simulink model "motor_ac"  (R2022b)
settings: Solver=VariableStepAuto  StartTime=0.0  StopTime=0.05  RelTol=1e-9  AbsTol=1e-9
values from neighbouring files (symbols this model uses):
  a1 = 1    [loop_sim.m]    (also in var_motor.m)
  a2 = 0.05    [loop_sim.m]    (also in sim_motor.m = a2s(i); var_motor.m)
  a3 = 0.02    [loop_sim.m]    (also in sim_motor.m = a3s(i); var_motor.m)
  Bm = 80e-6    (= 8e-05)    [loop_sim.m]    (also in var_motor.m)
  Jm = 40e-6    (= 4e-05)    [loop_sim.m]    (also in var_motor.m)
  Lls = 0.2e-3    (= 0.0002)    [loop_sim.m]    (also in var_motor.m)
  Lmb = 1.8e-3    (= 0.0018)    [loop_sim.m]    (also in var_motor.m)
  P = 4    [loop_sim.m]    (also in var_motor.m)
  psim = 0.1    [loop_sim.m]    (also in sim_motor.m = PSIs(i); var_motor.m)
  rs = 1    [loop_sim.m]    (also in sim_motor.m = RSs(i); var_motor.m)
  TL = 0.5    [loop_sim.m]    (also in var_motor.m = 0.1)
  TL0 = 0.5    [loop_sim.m]    (also in var_motor.m = 0.1)
  uM = 50    [loop_sim.m]    (also in var_motor.m)
settings Model: Creator=yodap  LastModifiedBy=andre
settings OptimizationCC: ReuseModelBlockBuffer=on

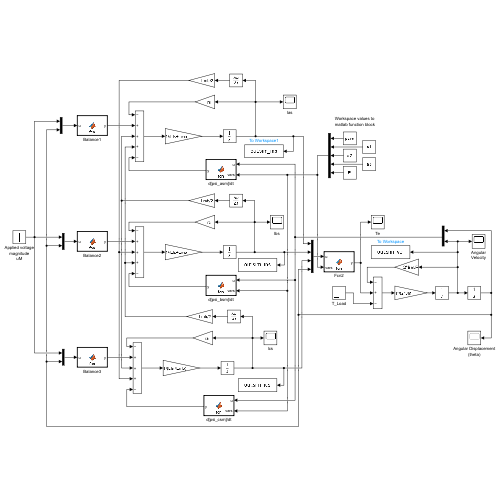
[thumbnail: Simulink's stored preview of the top-level diagram]
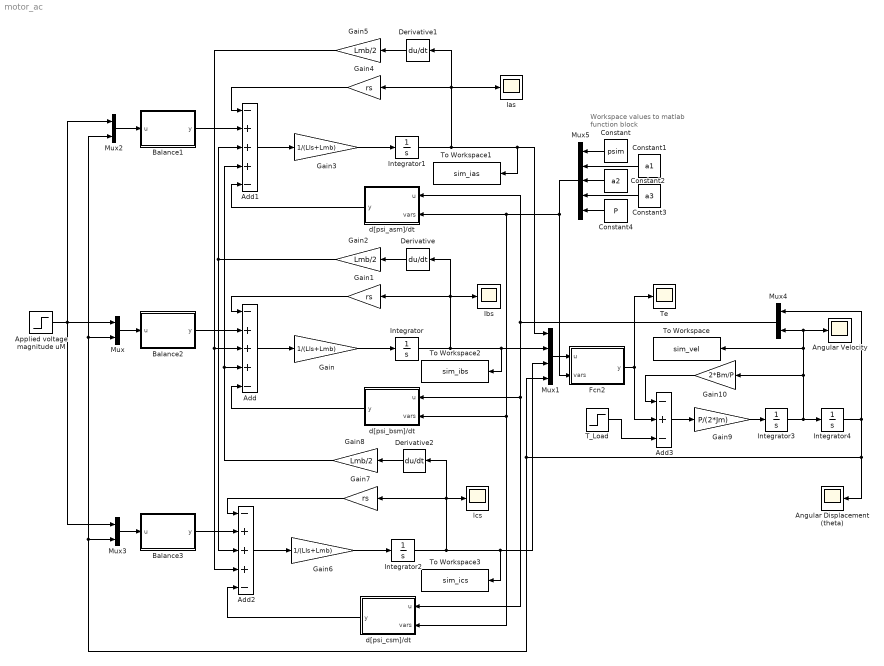
== system motor_ac ==
  note: Workspace values to
      | matlab function block
  Add : Sum  Inputs=-+++-
  Add1 : Sum  Inputs=-+++-
  Add2 : Sum  Inputs=-+++-
  Add3 : Sum  Inputs=-+-
  Angular Velocity : Scope
  Angular Displacement (theta) : Scope
  Applied voltage magnitude uM : Step  Time=0  After=uM  SampleTime=0
  Balance1 : MATLAB Function  TreatAsAtomicUnit=on
  Balance2 : MATLAB Function  TreatAsAtomicUnit=on
  Balance3 : MATLAB Function  TreatAsAtomicUnit=on
  Constant : Constant  Value=psim
  Constant1 : Constant  Value=a1
  Constant2 : Constant  Value=a2
  Constant3 : Constant  Value=a3
  Constant4 : Constant  Value=P
  Derivative : Derivative
  Derivative1 : Derivative
  Derivative2 : Derivative
  Fcn2 : MATLAB Function  TreatAsAtomicUnit=on
  Gain : Gain  Gain=1/(Lls+Lmb)
  Gain1 : Gain  Gain=rs
  Gain10 : Gain  Gain=2*Bm/P
  Gain2 : Gain  Gain=Lmb/2
  Gain3 : Gain  Gain=1/(Lls+Lmb)
  Gain4 : Gain  Gain=rs
  Gain5 : Gain  Gain=Lmb/2
  Gain6 : Gain  Gain=1/(Lls+Lmb)
  Gain7 : Gain  Gain=rs
  Gain8 : Gain  Gain=Lmb/2
  Gain9 : Gain  Gain=P/(2*Jm)
  Ias : Scope
  Ibs : Scope
  Integrator{,1..4} (5 alike) : Integrator
  Mux{,2..4} (4 alike) : Mux  Inputs=2
  Mux1 : Mux
  Mux5 : Mux  Inputs=5
  T_Load : Step  Time=0.025  Before=TL0  After=TL  SampleTime=0
  Te : Scope
  To Workspace : ToWorkspace  VariableName=sim_vel  SaveFormat=Timeseries  SampleTime=-1
  To Workspace1 : ToWorkspace  VariableName=sim_ias  SaveFormat=Timeseries  SampleTime=-1
  To Workspace2 : ToWorkspace  VariableName=sim_ibs  SaveFormat=Timeseries  SampleTime=-1
  To Workspace3 : ToWorkspace  VariableName=sim_ics  SaveFormat=Timeseries  SampleTime=-1
  d[psi_asm]/dt : MATLAB Function  TreatAsAtomicUnit=on
  d[psi_bsm]/dt : MATLAB Function  TreatAsAtomicUnit=on
  d[psi_csm]/dt : MATLAB Function  TreatAsAtomicUnit=on
  lcs : Scope
  wires:
  Mux/1 -> Balance2/1(u)
  Applied voltage magnitude uM/1 -> Mux3/1, Mux2/1, Mux/1
  Add/1 -> Gain/1
  Gain/1 -> Integrator/1
  Gain1/1 -> Add/1
  Integrator/1 -> To Workspace2/1, Mux1/2, Ibs/1, Gain1/1, Derivative/1
  Derivative/1 -> Gain2/1
  Gain3/1 -> Integrator1/1
  Add1/1 -> Gain3/1
  Gain4/1 -> Add1/1
  Derivative1/1 -> Gain5/1
  Integrator1/1 -> Gain4/1, Ias/1, Derivative1/1, To Workspace1/1, Mux1/1
  Gain2/1 -> Add2/3, Add1/3
  Balance1/1(y) -> Add1/2
  Mux2/1 -> Balance1/1(u)
  Derivative2/1 -> Gain8/1
  Integrator2/1 -> Derivative2/1, Gain7/1, lcs/1, To Workspace3/1, Mux1/3
  d[psi_csm]/dt/1(y) -> Add2/5
  Gain7/1 -> Add2/1
  Gain6/1 -> Integrator2/1
  Add2/1 -> Gain6/1
  Gain8/1 -> Add1/4, Add/4
  Gain5/1 -> Add2/4, Add/3
  T_Load/1 -> Add3/3
  Add3/1 -> Gain9/1
  Gain9/1 -> Integrator3/1
  Gain10/1 -> Add3/1
  Integrator3/1 -> Mux4/2, Angular Velocity/1, To Workspace/1, Gain10/1, Integrator4/1
  Mux4/1 -> d[psi_csm]/dt/1(u), d[psi_bsm]/dt/1(u), d[psi_asm]/dt/1(u)
  Integrator4/1 -> Mux2/2, Mux/2, Mux3/2, Mux1/4, Angular Displacement (theta)/1, Mux4/1
  Mux1/1 -> Fcn2/1(u)
  Fcn2/1(y) -> Te/1, Add3/2
  Balance2/1(y) -> Add/2
  Mux3/1 -> Balance3/1(u)
  Balance3/1(y) -> Add2/2
  d[psi_bsm]/dt/1(y) -> Add/5
  d[psi_asm]/dt/1(y) -> Add1/5
  Constant1/1 -> Mux5/2
  Constant2/1 -> Mux5/3
  Constant3/1 -> Mux5/4
  Constant/1 -> Mux5/1
  Mux5/1 -> Fcn2/2(vars), d[psi_csm]/dt/2(vars), d[psi_bsm]/dt/2(vars), d[psi_asm]/dt/2(vars)
  Constant4/1 -> Mux5/5

== matlab function motor_ac/Fcn2 ==
  data: u input; y output; vars input
function y = fcn(u,vars)

psim = vars(1);
a1 = vars(2);
a2 = vars(3);
a3 = vars(4);
P = vars(5);

y = P*psim*(u(1)*cos(u(4))*(a1+3*a2*(sin(u(4)))^2+5*a3*(sin(u(4)))^4)+u(2)*cos(u(4)+2*pi/3)*(a1+3*a2*(sin(u(4)+2*pi/3))^2+5*a3*(sin(u(4)+2*pi/3))^4)+u(3)*cos(u(4)-2*pi/3)*(a1+3*a2*(sin(u(4)-2*pi/3))^2+5*a3*(sin(u(4)-2*pi/3))^4))/2;
% y = P*psim*(u(1)*cos(u(4))*(a1+3*a2*(sin(u(4)))^2+5*a3*(sin(u(4)))^4)+u(2)*cos(u(4)+pi/6)*(a1+3*a2*(sin(u(4)+pi/6))^2+5*a3*(sin(u(4)+pi/6))^4)+u(3)*cos(u(4)-pi/3)*(a1+3*a2*(sin(u(4)-pi/3))^2+5*a3*(sin(u(4)-pi/3))^4))/2; % unbalanced

== matlab function motor_ac/Balance2 ==
  data: u input; y output
function y = fcn(u)

y = u(1)*cos(u(2)+2*pi/3);

== matlab function motor_ac/Balance3 ==
  data: u input; y output
function y = fcn(u)

y = u(1)*cos(u(2)-2*pi/3);

== matlab function motor_ac/d[psi_asm]//dt ==
  data: u input; y output; vars input
function y = fcn(u,vars)

psim = vars(1);
a1 = vars(2);
a2 = vars(3);
a3 = vars(4);

y = psim*(u(2)*cos(u(1))*(a1+3*a2*(sin(u(1)))^2+5*a3*(sin(u(1)))^4));

== matlab function motor_ac/d[psi_bsm]//dt ==
  data: u input; y output; vars input
function y = fcn(u,vars)

psim = vars(1);
a1 = vars(2);
a2 = vars(3);
a3 = vars(4);

y = psim*(u(2)*cos(u(1)+2*pi/3)*(a1+3*a2*(sin(u(1)+2*pi/3))^2+5*a3*(sin(u(1)+2*pi/3))^4));
% y = psim*(u(2)*cos(u(1)+pi/6)*(a1+3*a2*(sin(u(1)+pi/6))^2+5*a3*(sin(u(1)+pi/6))^4)); % unbalanced

== matlab function motor_ac/d[psi_csm]//dt ==
  data: u input; y output; vars input
function y = fcn(u,vars)

psim = vars(1);
a1 = vars(2);
a2 = vars(3);
a3 = vars(4);

y = psim*(u(2)*cos(u(1)-2*pi/3)*(a1+3*a2*(sin(u(1)-2*pi/3))^2+5*a3*(sin(u(1)-2*pi/3))^4));
% y = psim*(u(2)*cos(u(1)-pi/3)*(a1+3*a2*(sin(u(1)-pi/3))^2+5*a3*(sin(u(1)-pi/3))^4)); % unbalanced

== matlab function motor_ac/Balance1 ==
  data: u input; y output
function y = fcn(u)

y = u(1)*cos(u(2));
